simulink model "Examen_Observabilidad_Feedback_v2"  (R2022a)
settings: Solver=VariableStepAuto  StartTime=0.0  StopTime=2  RelTol=1e-3
values from neighbouring files (symbols this model uses):
  A = [22 7 11;-64 -19 -26;-26 -8 -16]    [untitled2.m]
  B = [2;-4;-3]    [untitled2.m]
  K = cell(1,NoEqns)    [untitled2.m]
undefined symbols (not defined in the file or in its folder): C, L, Ueq, x0, x0b
settings Model: Creator=fernando  LastModifiedBy=fernando

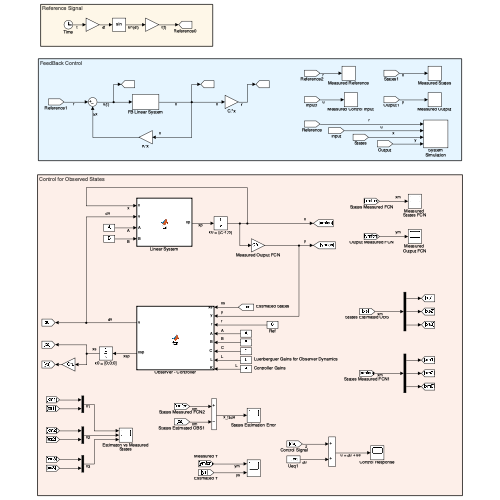
[thumbnail: Simulink's stored preview of the top-level diagram]
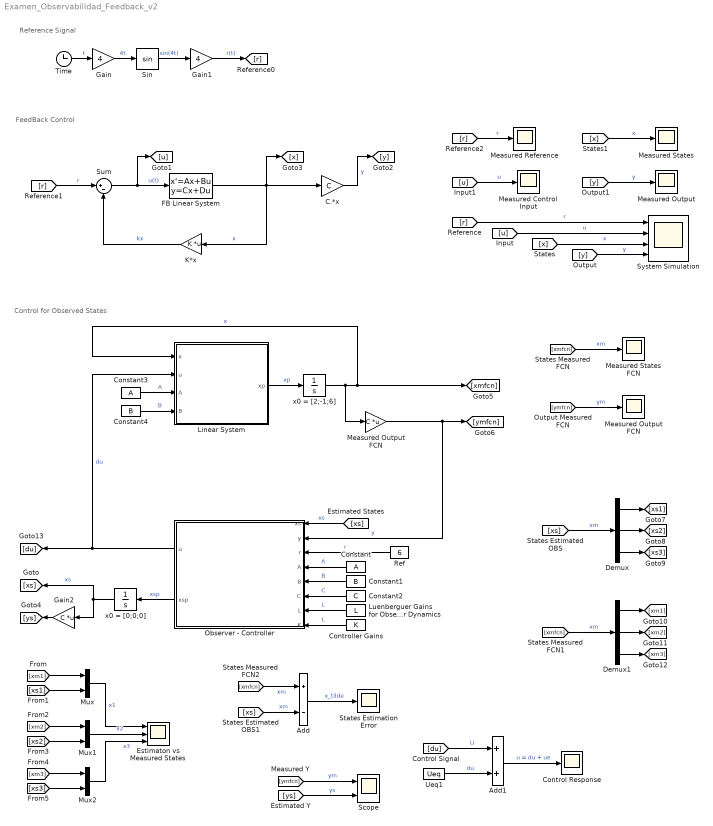
== system Examen_Observabilidad_Feedback_v2 ==
  note: Control for Observed States
  note: FeedBack Control
  note: Reference Signal
  Add : Sum  Inputs=+-
  Add1 : Sum
  C.*x : Gain  Gain=C
  Constant : Constant  Value=A  VectorParams1D=off
  Constant1 : Constant  Value=B  VectorParams1D=off
  Constant2 : Constant  Value=C  VectorParams1D=off
  Constant3 : Constant  Value=A
  Constant4 : Constant  Value=B
  Control Response : Scope
  Controller Gains : Constant  Value=K  VectorParams1D=off
  Demux : Demux  Outputs=3
  Demux1 : Demux  Outputs=3
  Estimaton vs Measured States : Scope  NumInputPorts=3
  FB Linear System : StateSpace  A=A  B=B  C=eye(3)  D=zeros(3,1)  InitialCondition=x0
  Gain : Gain  Gain=4
  Gain1 : Gain  Gain=4
  Gain2 : Gain  Gain=C  Multiplication=Matrix(K*u)
  K*x : Gain  Gain=K  Multiplication=Matrix(K*u)
  Linear System : MATLAB Function  TreatAsAtomicUnit=on
  Luenberguer Gains for Observer Dynamics : Constant  Value=L  VectorParams1D=off
  Measured Output FCN : Scope
  Measured States FCN : Scope
  Measured Control Input : Scope
  Measured Output : Scope
  Measured Output FCN : Gain  Gain=C  Multiplication=Matrix(K*u)
  Measured Reference : Scope
  Measured States : Scope
  Mux : Mux  Inputs=2
  Mux1 : Mux  Inputs=2
  Mux2 : Mux  Inputs=2
  Observer - Controller : MATLAB Function  TreatAsAtomicUnit=on
  Ref : Constant  Value=6  VectorParams1D=off
  Scope : Scope  NumInputPorts=2
  Sin : Trigonometry
  States Estimation Error : Scope
  Sum : Sum  Inputs=|+-
  System Simulation : Scope  NumInputPorts=4
  Time : Clock
  Ueq1 : Constant  Value=Ueq  VectorParams1D=off
  x0 = [0;0;0] : Integrator  InitialCondition=x0b
  x0 = [2;-1;6] : Integrator  InitialCondition=x0
  wires:
  FB Linear System/1 -> [x], K*x/1, C.*x/1  "x"
  Time/1 -> Gain/1  "t"
  Gain/1 -> Sin/1  "4t"
  Sin/1 -> Gain1/1  "sin(4t)"
  C.*x/1 -> [y]  "y"
  K*x/1 -> Sum/2  "kx"
  Sum/1 -> FB Linear System/1, [u]  "u(t)"
  [r] -> System Simulation/1  "r"
  [u] -> System Simulation/2  "u"
  [x] -> System Simulation/3  "x"
  [y] -> System Simulation/4  "y"
  Observer - Controller/2(xsp) -> x0 = [0;0;0]/1  "xsp"
  Ref/1 -> Observer - Controller/3(r)  "r"
  Constant2/1 -> Observer - Controller/6(C)  "C"
  Constant1/1 -> Observer - Controller/5(B)  "B"
  Constant/1 -> Observer - Controller/4(A)  "A"
  Luenberguer Gains for Observer Dynamics/1 -> Observer - Controller/7(L)  "L"
  Measured Output FCN/1 -> Observer - Controller/2(y), [ymfcn]  "y"
  Gain1/1 -> [r]  "r(t)"
  [r] -> Sum/1  "r"
  [r] -> Measured Reference/1  "r"
  [x] -> Measured States/1  "x"
  [y] -> Measured Output/1  "y"
  [u] -> Measured Control Input/1  "u"
  x0 = [0;0;0]/1 -> [xs], Gain2/1  "xs"
  [xs] -> Observer - Controller/1(xs)  "xs"
  Constant3/1 -> Linear System/3(A)  "A"
  Constant4/1 -> Linear System/4(B)  "B"
  Linear System/1(xp) -> x0 = [2;-1;6]/1  "xp"
  Observer - Controller/1(u) -> [du], Linear System/2(u)  "du"
  [xmfcn] -> Measured States FCN/1  "xm"
  [ymfcn] -> Measured Output FCN/1  "ym"
  x0 = [2;-1;6]/1 -> Measured Output FCN/1, Linear System/1(x), [xmfcn]  "x"
  [xs] -> Demux/1  "xm"
  [xmfcn] -> Demux1/1  "xm"
  Demux/1 -> [xs1]
  Demux/3 -> [xs3]
  Demux/2 -> [xs2]
  Demux1/2 -> [xm2]
  Demux1/3 -> [xm3]
  Demux1/1 -> [xm1]
  [xmfcn] -> Add/1  "xm"
  [xs] -> Add/2  "xm"
  Add/1 -> States Estimation Error/1  "x_tilde"
  [xm1] -> Mux/1
  [xs1] -> Mux/2
  [xm2] -> Mux1/1
  [xs2] -> Mux1/2
  [xm3] -> Mux2/1
  [xs3] -> Mux2/2
  Mux1/1 -> Estimaton vs Measured States/2  "x2"
  Mux/1 -> Estimaton vs Measured States/1  "x1"
  Mux2/1 -> Estimaton vs Measured States/3  "x3"
  Gain2/1 -> [ys]
  [ymfcn] -> Scope/1  "ym"
  [ys] -> Scope/2  "ys"
  Controller Gains/1 -> Observer - Controller/8(K)  "L"
  [du] -> Add1/1  "U"
  Add1/1 -> Control Response/1  "u = du + ue"
  Ueq1/1 -> Add1/2  "du"

== matlab function Examen_Observabilidad_Feedback_v2/Linear System ==
  data: x input; xp output; u input; A input; B input
function xp = fcn(x,u,A,B)

xp = A*x + B*u;

== matlab function Examen_Observabilidad_Feedback_v2/Observer - Controller ==
  data: u output; xs input; y input; xsp output; r input; A input; B input; C input; L input; K input
function [u,xsp] = fcn(xs,y,r,A,B,C,L,K)

xsp = (A -L*C -B*K)*xs + B*r + L*(y);

u = -K*xs + r;
